simulink model "simulated_physical_reactor_v4_isolated"  (R2023a)
settings: Solver=FixedStepAuto  StartTime=0.0  StopTime=500  FixedStep=ts  RelTol=1e-3
values from neighbouring files (symbols this model uses):
  actionDelay = 10    [MainCode.m]
  buffer = 10    [MainCode.m]
  C0_attack_c = 0    [MainCode.m]
  C0_noise = 1    [MainCode.m]
  C0_post_attack = 0    [MainCode.m]
  C0_post_attack_val = -.25    (= -0.25)    [MainCode.m]
  Ccell0 = cell0 / v_cell    (= 15384.6153846)    [MainCode.m]
  CG0 = 185    [MainCode.m]
  CG_attack_c = 55    [MainCode.m]
  CG_attack_time = 175    [MainCode.m]
  CG_fake_failure = 0    [MainCode.m]
  CG_fake_failure_noise = 8    [MainCode.m]
  CG_increase_b = 0    [MainCode.m]
  CG_increase_rate = 2    [MainCode.m]
  cg_noGrowth = 10    [MainCode.m]
  CG_noise = 1    [MainCode.m]
  CG_post_attack = 1    [MainCode.m]
  CG_post_attack_val = .25    (= 0.25)    [MainCode.m]
  CG_ramp_attack = 1    [MainCode.m]
  CG_ramp_time = 125    [MainCode.m]
  CG_target = 50    [MainCode.m]
  CM = 4    [MainCode.m]
  CO0 = .245    (= 0.245)    [MainCode.m]
  CO_attack_time = 80    [MainCode.m]
  CO_fake_failure = 0    [MainCode.m]
  CO_fake_failure_mean = .08    (= 0.08)    [MainCode.m]
  CO_fake_failure_noise = .005    (= 0.005)    [MainCode.m]
  CO_ramp_attack = 0    [MainCode.m]
  CO_ramp_time = 100    [MainCode.m]
  count_thresh = 3    [MainCode.m]
  F_fresh_max = 25    [MainCode.m]
  F_net = F_fresh_start + F_recycle_start    (= 334.8)    [MainCode.m]
  flowrateNoiseActive = 0    [MainCode.m]
  flowrateNoiseVal = 0.5 / 100    (= 0.005)    [MainCode.m]
  fresh_attack = 0    [MainCode.m]
  fresh_attack_time = 70    [MainCode.m]
  fresh_attack_val = .1    (= 0.1)    [MainCode.m]
  freshPump_fail_time = 30    [MainCode.m]
  freshPump_failure = 0    [MainCode.m]
  freshPump_response_increases = 2    [MainCode.m]
  freshPump_response_window = 10    [MainCode.m]
  g_failure_start_t = 80    [MainCode.m]
  g_fault_wait_time = 10    [MainCode.m]
  g_flowrate_control_windowsize = 10    [MainCode.m]
  g_lownoise_val = 1.25    [MainCode.m]
  g_numpoints_fail = g_standdev_window_size+1    (= 16)    [MainCode.m]
  g_numpoints_low = 4    [MainCode.m]
  g_prob_arraylen = 15    [MainCode.m]
  g_prob_count = 6    [MainCode.m]
  g_prob_thresh = .45    (= 0.45)    [MainCode.m]
  g_standdev_window_size = 15    [MainCode.m]
  g_standev_tol = 7    [MainCode.m]
  glucose_fail_noise = 10    [MainCode.m]
  glucosesensor_failure = 0    [MainCode.m]
  lowConc_controller_onState = 1    [MainCode.m]
  mean_noise_C0 = 0    [MainCode.m]
  mean_noise_CG = 0    [MainCode.m]
  mu_max = 0.0251    [MainCode.m]
  n_size = t_window/ts    (= 2.5)    [MainCode.m]
  n_size_CG = n_size    (= 2.5)    [MainCode.m]
  o2_alpha = .20    (= 0.2)    [MainCode.m]
  o2_fail_mean = .008    (= 0.008)    [MainCode.m]
  o2_fail_noise = .005    (= 0.005)    [MainCode.m]
  o2_fail_time = 50    [MainCode.m]
  o2_fault_halfrange = .01    (= 0.01)    [MainCode.m]
  o2_fault_numpoints = 5    [MainCode.m]
  o2_lownoise_val = .0008    (= 0.0008)    [MainCode.m]
  o2_movingaverage_window = 10    [MainCode.m]
  o2_numpoints_low = 6    [MainCode.m]
  o2_prob_arraylen = 10    [MainCode.m]
  o2_prob_count = 6    [MainCode.m]
  o2_prob_thresh = .45    (= 0.45)    [MainCode.m]
  o2sensor_failure = 0    [MainCode.m]
  OCR = 2.8e-11    [MainCode.m]
  p_thresh = .4    (= 0.4)    [MainCode.m]
  rec_attack = 0    [MainCode.m]
  rec_attack_time = 50    [MainCode.m]
  rec_attack_val = 120    [MainCode.m]
  recPump_drop_val = .02    (= 0.02)    [MainCode.m]
  recPump_fail_time = 30    [MainCode.m]
  recPump_failure = 0    [MainCode.m]
  recPump_rollingavg_samples_buildup = 10    [MainCode.m]
  recPump_smallDrop_size = 0.006    [MainCode.m]
  stdev_noise_C0 = .002    (= 0.002)    [MainCode.m]
  stdev_noise_CG = 3.5    [MainCode.m]
  t_crit_CG = .7    (= 0.7)    [MainCode.m]
  ts = 1    [MainCode.m]
  V = 65.0    (= 65)    [MainCode.m]
  v_cell = 65    [MainCode.m]
  YGC = 155 * 10^-6    (= 0.000155)    [MainCode.m]
undefined symbols (not defined in the file or in its folder): DiscIntNeverNeededParam, recPump_numDrops_waitTime, recPump_rollingavg_numDrops
libraries: simulink x16, sldrtlib x11, dspstat3 x8, aerolibanimutils x1
(part 2 of 3)

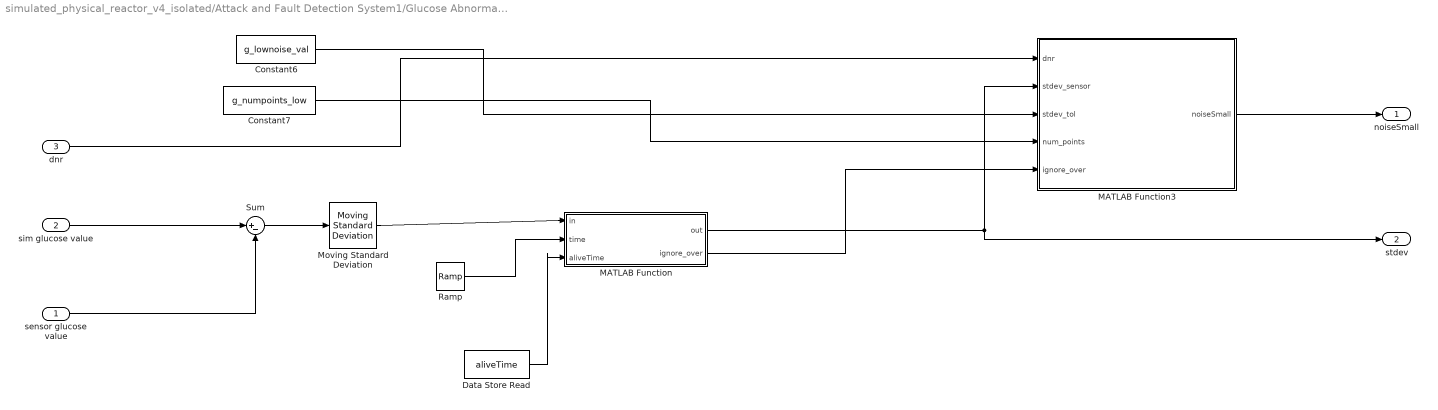
== system simulated_physical_reactor_v4_isolated/Attack and Fault Detection System1/Glucose Abnormally Low Noise Detection ==
  sensor glucose value : Inport
  sim glucose value : Inport  Port=2
  dnr : Inport  Port=3
  Constant6 : Constant  Value=g_lownoise_val
  Constant7 : Constant  Value=g_numpoints_low
  Data Store Read : DataStoreRead  DataStoreName=aliveTime  IndexOptions=Index vector (dialog)  Indices=1  OutputSizes=1
  MATLAB Function : MATLAB Function  TreatAsAtomicUnit=on
  MATLAB Function3 : MATLAB Function  TreatAsAtomicUnit=on
  Moving Standard Deviation : dspstat3/Moving Standard Deviation  Method=Sliding window  ForgettingFactorPort=off  SpecifyWindowLength=on  WindowLength=g_standdev_window_size  OverlapLength=g_standdev_window_size-1  AllowArbitraryInputLength=off  ForgettingFactor=0.9  SimulateUsing=Code generation
  Ramp : simulink/Sources/Ramp  slope=1  start=0  InitialOutput=0
  Sum : Sum  Inputs=|+-
  noiseSmall : Outport
  stdev : Outport  Port=2
  wires:
  MATLAB Function3/1(noiseSmall) -> noiseSmall/1
  Sum/1 -> Moving Standard Deviation/1
  Moving Standard Deviation/1 -> MATLAB Function/1(in)
  Ramp/1 -> MATLAB Function/2(time)
  sim glucose value/1 -> Sum/1
  MATLAB Function/1(out) -> MATLAB Function3/2(stdev_sensor), stdev/1
  sensor glucose value/1 -> Sum/2
  Constant6/1 -> MATLAB Function3/3(stdev_tol)
  Constant7/1 -> MATLAB Function3/4(num_points)
  MATLAB Function/2(ignore_over) -> MATLAB Function3/5(ignore_over)
  dnr/1 -> MATLAB Function3/1(dnr)
  Data Store Read/1 -> MATLAB Function/3(aliveTime)

== system simulated_physical_reactor_v4_isolated/Attack and Fault Detection System1/Glucose Deviation Detection ==
  Simulated g value : Inport
  Sensor g value : Inport  Port=2
  dnr : Inport  Port=3
  Constant : Constant  Value=g_prob_arraylen
  Constant1 : Constant  Value=g_prob_thresh
  Constant2 : Constant  Value=g_prob_count
  MATLAB Function : MATLAB Function  TreatAsAtomicUnit=on
  MATLAB Function1 : MATLAB Function  TreatAsAtomicUnit=on
  Moving Standard Deviation : dspstat3/Moving Standard Deviation  Method=Sliding window  ForgettingFactorPort=off  SpecifyWindowLength=on  WindowLength=g_standdev_window_size  OverlapLength=g_standdev_window_size-1  AllowArbitraryInputLength=off  ForgettingFactor=0.9  SimulateUsing=Code generation
  Sum : Sum  Inputs=|+-
  isDeviated : Outport
  likelihood : Outport  Port=2
  wires:
  Moving Standard Deviation/1 -> MATLAB Function/3(std_dev)
  MATLAB Function/1(likelihood) -> likelihood/1, MATLAB Function1/2(prob)
  Simulated g value/1 -> Sum/2
  Constant/1 -> MATLAB Function/4(g_prob_arraylen)
  Sensor g value/1 -> Moving Standard Deviation/1, Sum/1
  Sum/1 -> MATLAB Function/2(new_sens_value)
  MATLAB Function1/1(isDeviated) -> isDeviated/1
  Constant1/1 -> MATLAB Function1/3(thresh)
  Constant2/1 -> MATLAB Function1/4(thresh_count)
  dnr/1 -> MATLAB Function1/1(dnr), MATLAB Function/1(dnr)

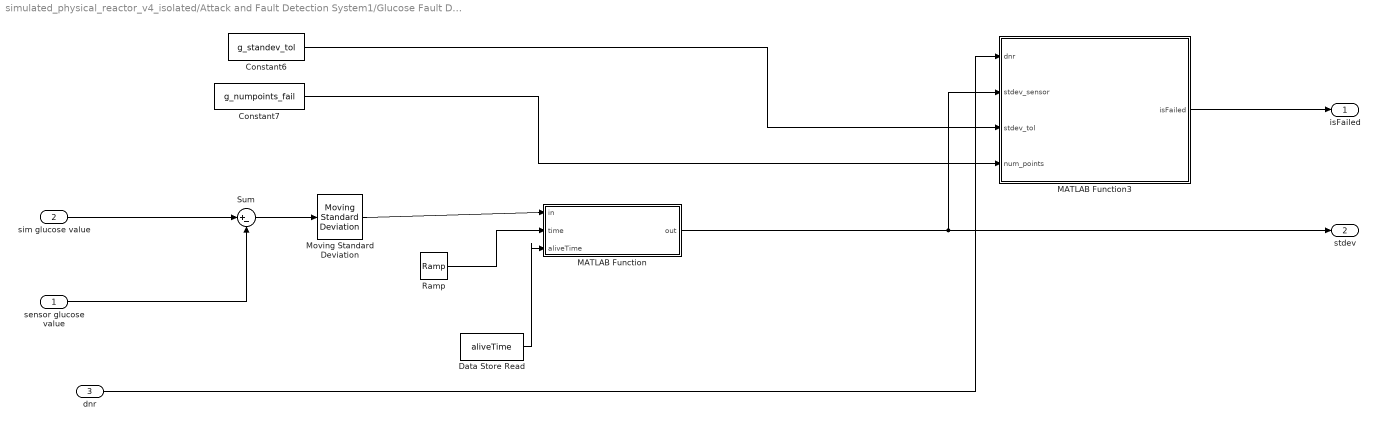
== system simulated_physical_reactor_v4_isolated/Attack and Fault Detection System1/Glucose Fault Detection ==
  sensor glucose value : Inport
  sim glucose value : Inport  Port=2
  dnr : Inport  Port=3
  Constant6 : Constant  Value=g_standev_tol
  Constant7 : Constant  Value=g_numpoints_fail
  Data Store Read : DataStoreRead  DataStoreName=aliveTime  IndexOptions=Index vector (dialog)  Indices=1  OutputSizes=1
  MATLAB Function : MATLAB Function  TreatAsAtomicUnit=on
  MATLAB Function3 : MATLAB Function  TreatAsAtomicUnit=on
  Moving Standard Deviation : dspstat3/Moving Standard Deviation  Method=Sliding window  ForgettingFactorPort=off  SpecifyWindowLength=on  WindowLength=g_standdev_window_size  OverlapLength=g_standdev_window_size-1  AllowArbitraryInputLength=off  ForgettingFactor=0.9  SimulateUsing=Code generation
  Ramp : simulink/Sources/Ramp  slope=1  start=0  InitialOutput=0
  Sum : Sum  Inputs=|+-
  isFailed : Outport
  stdev : Outport  Port=2
  wires:
  sim glucose value/1 -> Sum/1
  sensor glucose value/1 -> Sum/2
  MATLAB Function/1(out) -> stdev/1, MATLAB Function3/2(stdev_sensor)
  Sum/1 -> Moving Standard Deviation/1
  Moving Standard Deviation/1 -> MATLAB Function/1(in)
  Constant7/1 -> MATLAB Function3/4(num_points)
  Constant6/1 -> MATLAB Function3/3(stdev_tol)
  Ramp/1 -> MATLAB Function/2(time)
  MATLAB Function3/1(isFailed) -> isFailed/1
  dnr/1 -> MATLAB Function3/1(dnr)
  Data Store Read/1 -> MATLAB Function/3(aliveTime)

== system simulated_physical_reactor_v4_isolated/Attack and Fault Detection System1/Oxygen Abnormally Low Noise Detection1 ==
  sensor o2 value : Inport
  sim o2 value : Inport  Port=2
  dnr : Inport  Port=3
  Constant6 : Constant  Value=o2_lownoise_val
  Constant7 : Constant  Value=o2_numpoints_low
  Data Store Read : DataStoreRead  DataStoreName=aliveTime  IndexOptions=Index vector (dialog)  Indices=1  OutputSizes=1
  MATLAB Function : MATLAB Function  TreatAsAtomicUnit=on
  MATLAB Function3 : MATLAB Function  TreatAsAtomicUnit=on
  Moving Standard Deviation : dspstat3/Moving Standard Deviation  Method=Sliding window  ForgettingFactorPort=off  SpecifyWindowLength=on  WindowLength=g_standdev_window_size  OverlapLength=g_standdev_window_size-1  AllowArbitraryInputLength=off  ForgettingFactor=0.9  SimulateUsing=Code generation
  Ramp : simulink/Sources/Ramp  slope=1  start=0  InitialOutput=0
  Sum : Sum  Inputs=|+-
  noiseSmall : Outport
  stdev : Outport  Port=2
  wires:
  MATLAB Function3/1(noiseSmall) -> noiseSmall/1
  Sum/1 -> Moving Standard Deviation/1
  Moving Standard Deviation/1 -> MATLAB Function/1(in)
  Ramp/1 -> MATLAB Function/2(time)
  sim o2 value/1 -> Sum/1
  MATLAB Function/1(out) -> MATLAB Function3/2(stdev_sensor), stdev/1
  sensor o2 value/1 -> Sum/2
  Constant6/1 -> MATLAB Function3/3(stdev_tol)
  Constant7/1 -> MATLAB Function3/4(num_points)
  MATLAB Function/2(ignore_over) -> MATLAB Function3/5(ignore_over)
  dnr/1 -> MATLAB Function3/1(dnr)
  Data Store Read/1 -> MATLAB Function/3(aliveTime)

== system simulated_physical_reactor_v4_isolated/Attack and Fault Detection System1/Oxygen Deviation Detection1 ==
  Simulated o2 value : Inport
  Sensor o2 value : Inport  Port=2
  dnr : Inport  Port=3
  Constant : Constant  Value=o2_prob_arraylen
  Constant1 : Constant  Value=o2_prob_thresh
  Constant2 : Constant  Value=o2_prob_count
  MATLAB Function : MATLAB Function  TreatAsAtomicUnit=on
  MATLAB Function1 : MATLAB Function  TreatAsAtomicUnit=on
  Moving Standard Deviation : dspstat3/Moving Standard Deviation  Method=Sliding window  ForgettingFactorPort=off  SpecifyWindowLength=on  WindowLength=g_standdev_window_size  OverlapLength=g_standdev_window_size-1  AllowArbitraryInputLength=off  ForgettingFactor=0.9  SimulateUsing=Code generation
  Sum : Sum  Inputs=|+-
  isDeviated : Outport
  likelihood : Outport  Port=2
  wires:
  Moving Standard Deviation/1 -> MATLAB Function/3(std_dev)
  MATLAB Function/1(likelihood) -> likelihood/1, MATLAB Function1/2(prob)
  Simulated o2 value/1 -> Sum/2
  Constant/1 -> MATLAB Function/4(o2_prob_arraylen)
  Sensor o2 value/1 -> Moving Standard Deviation/1, Sum/1
  Sum/1 -> MATLAB Function/2(new_sens_value)
  MATLAB Function1/1(isDeviated) -> isDeviated/1
  Constant1/1 -> MATLAB Function1/3(thresh)
  Constant2/1 -> MATLAB Function1/4(thresh_count)
  dnr/1 -> MATLAB Function1/1(dnr), MATLAB Function/1(dnr)

== system simulated_physical_reactor_v4_isolated/Attack and Fault Detection System1/Oxygen Sensor Failure Detection ==
  o2_sensor : Inport
  dnr : Inport  Port=2
  Constant : Constant  Value=o2_fail_mean
  Constant2 : Constant  Value=o2_fault_halfrange
  Constant3 : Constant  Value=o2_fault_numpoints
  MATLAB Function : MATLAB Function  TreatAsAtomicUnit=on
  MATLAB Function1 : MATLAB Function  TreatAsAtomicUnit=on
  MATLAB Function2 : MATLAB Function  TreatAsAtomicUnit=on
  isFailed : Outport
  o2Distrubed : Outport  Port=2
  wires:
  Constant2/1 -> MATLAB Function2/4(half_range)
  Constant3/1 -> MATLAB Function2/5(num_points)
  Constant/1 -> MATLAB Function2/3(fail_val)
  o2_sensor/1 -> MATLAB Function2/2(o2_sensor)
  MATLAB Function2/1(isFailed) -> MATLAB Function/5(isFailed_begin), MATLAB Function1/1(isFailed)
  MATLAB Function1/1(o2_fault) -> isFailed/1
  MATLAB Function1/2(o2_disturb) -> o2Distrubed/1
  MATLAB Function/1(isFlat) -> MATLAB Function1/2(isFlat)
  dnr/1 -> MATLAB Function2/1(dnr)

== system simulated_physical_reactor_v4_isolated/Attack and Fault Detection System1/Recycle Pump Fault Detection ==
  oxygen sensor : Inport
  dnr : Inport  Port=2
  net flowrate commanded : Inport  Port=3
  Constant : Constant  Value=recPump_drop_val
  Constant1 : Constant  Value=recPump_numDrops_waitTime
  Constant2 : Constant  Value=recPump_rollingavg_numDrops
  Constant3 : Constant  Value=recPump_rollingavg_samples_buildup
  Constant4 : Constant  Value=recPump_smallDrop_size
  MATLAB Function : MATLAB Function  TreatAsAtomicUnit=on
  noRecycleResponse : Outport
  delta_o2 : Outport  Port=2
  rolling_avg_o2 : Outport  Port=3
  wires:
  net flowrate commanded/1 -> MATLAB Function/2(new_flowrate_commanded)
  MATLAB Function/1(RecyclePumpFail) -> noRecycleResponse/1
  oxygen sensor/1 -> MATLAB Function/3(oxygen_sensor)
  Constant/1 -> MATLAB Function/8(large_drop_val)
  Constant1/1 -> MATLAB Function/6(rolling_avg_samples_wait)
  Constant4/1 -> MATLAB Function/7(o2_rollavg_drop_spec)
  Constant2/1 -> MATLAB Function/5(numDrops)
  Constant3/1 -> MATLAB Function/4(samples_to_wait)
  MATLAB Function/2(delta_o2_out) -> delta_o2/1
  MATLAB Function/3(rolling_avg_out) -> rolling_avg_o2/1
  dnr/1 -> MATLAB Function/1(dnr)

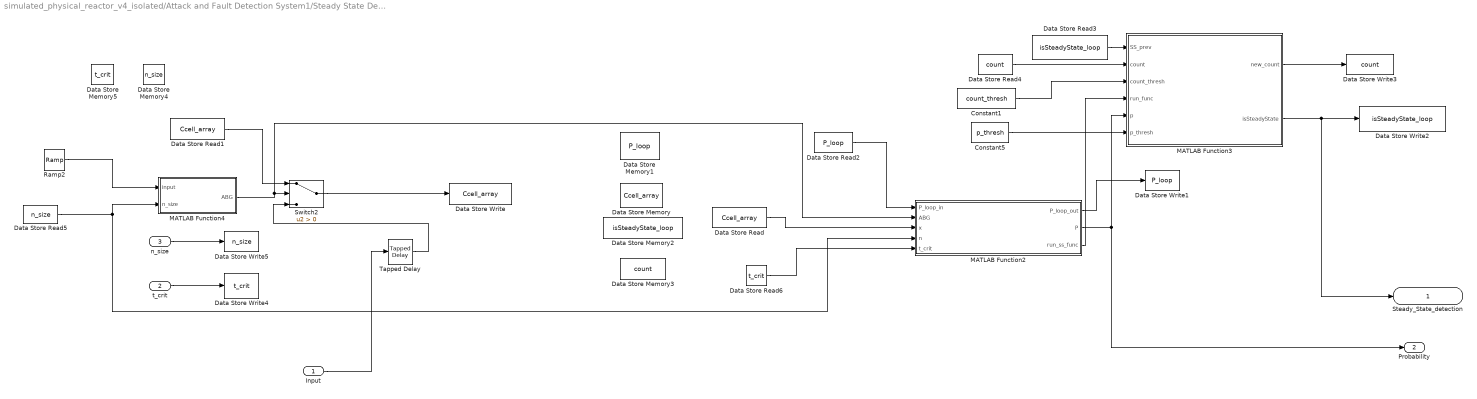
== system simulated_physical_reactor_v4_isolated/Attack and Fault Detection System1/Steady State Detection System1 ==
  Input : Inport
  t_crit : Inport  Port=2
  n_size : Inport  Port=3
  Constant1 : Constant  Value=count_thresh
  Constant5 : Constant  Value=p_thresh
  Data Store Memory : DataStoreMemory  DataStoreName=Ccell_array  ReadBeforeWriteMsg=warning  WriteAfterWriteMsg=warning  WriteAfterReadMsg=warning  InitialValue=zeros(1,n_size)  ShowAdditionalParam=off  OutDataTypeStr=double
  Data Store Memory1 : DataStoreMemory  DataStoreName=P_loop  ReadBeforeWriteMsg=warning  WriteAfterWriteMsg=warning  WriteAfterReadMsg=warning  ShowAdditionalParam=off
  Data Store Memory2 : DataStoreMemory  DataStoreName=isSteadyState_loop  ReadBeforeWriteMsg=warning  WriteAfterWriteMsg=warning  WriteAfterReadMsg=warning  ShowAdditionalParam=off
  Data Store Memory3 : DataStoreMemory  DataStoreName=count  ReadBeforeWriteMsg=warning  WriteAfterWriteMsg=warning  WriteAfterReadMsg=warning  ShowAdditionalParam=off
  Data Store Memory4 : DataStoreMemory  DataStoreName=n_size  ReadBeforeWriteMsg=warning  WriteAfterWriteMsg=warning  WriteAfterReadMsg=warning  ShowAdditionalParam=off
  Data Store Memory5 : DataStoreMemory  DataStoreName=t_crit  ReadBeforeWriteMsg=warning  WriteAfterWriteMsg=warning  WriteAfterReadMsg=warning  ShowAdditionalParam=off
  Data Store Read : DataStoreRead  DataStoreName=Ccell_array  IndexOptions=Index vector (dialog)  Indices=1  OutputSizes=1
  Data Store Read1 : DataStoreRead  DataStoreName=Ccell_array  IndexOptions=Index vector (dialog)  Indices=1  OutputSizes=1
  Data Store Read2 : DataStoreRead  DataStoreName=P_loop  IndexOptions=Index vector (dialog)  Indices=1  OutputSizes=1
  Data Store Read3 : DataStoreRead  DataStoreName=isSteadyState_loop  IndexOptions=Index vector (dialog)  Indices=1  OutputSizes=1
  Data Store Read4 : DataStoreRead  DataStoreName=count  IndexOptions=Index vector (dialog)  Indices=1  OutputSizes=1
  Data Store Read5 : DataStoreRead  DataStoreName=n_size  IndexOptions=Index vector (dialog)  Indices=1  OutputSizes=1
  Data Store Read6 : DataStoreRead  DataStoreName=t_crit  IndexOptions=Index vector (dialog)  Indices=1  OutputSizes=1
  Data Store Write : DataStoreWrite  DataStoreName=Ccell_array  IndexOptions=Index vector (dialog)  Indices=1  OutputSizes=1
  Data Store Write1 : DataStoreWrite  DataStoreName=P_loop  IndexOptions=Index vector (dialog)  Indices=1  OutputSizes=1
  Data Store Write2 : DataStoreWrite  DataStoreName=isSteadyState_loop  IndexOptions=Index vector (dialog)  Indices=1  OutputSizes=1
  Data Store Write3 : DataStoreWrite  DataStoreName=count  IndexOptions=Index vector (dialog)  Indices=1  OutputSizes=1
  Data Store Write4 : DataStoreWrite  DataStoreName=t_crit  IndexOptions=Index vector (dialog)  Indices=1  OutputSizes=1
  Data Store Write5 : DataStoreWrite  DataStoreName=n_size  IndexOptions=Index vector (dialog)  Indices=1  OutputSizes=1
  MATLAB Function2 : MATLAB Function  TreatAsAtomicUnit=on
  MATLAB Function3 : MATLAB Function  TreatAsAtomicUnit=on
  MATLAB Function4 : MATLAB Function  TreatAsAtomicUnit=on
  Ramp2 : simulink/Sources/Ramp  slope=1/ts  start=0  InitialOutput=0
  Switch2 : Switch  Criteria=u2 > Threshold  SaturateOnIntegerOverflow=off  InputSameDT=off
  Tapped Delay : simulink/Discrete/Tapped Delay  vinit=0.0  samptime=-1  NumDelays=n_size  DelayOrder=Oldest  includeCurrent=off
  Steady_State_detection : Outport
  Probability : Outport  Port=2
  wires:
  MATLAB Function3/2(isSteadyState) -> Steady_State_detection/1, Data Store Write2/1
  MATLAB Function2/1(P_loop_out) -> Data Store Write1/1
  Data Store Read2/1 -> MATLAB Function2/1(P_loop_in)
  Input/1 -> Tapped Delay/1
  Data Store Read4/1 -> MATLAB Function3/2(count)
  Data Store Read1/1 -> Switch2/1
  MATLAB Function2/2(P) -> Probability/1, MATLAB Function3/5(p)
  Constant5/1 -> MATLAB Function3/6(p_thresh)
  Data Store Read5/1 -> MATLAB Function4/2(n_size), MATLAB Function2/4(n)
  MATLAB Function3/1(new_count) -> Data Store Write3/1
  Ramp2/1 -> MATLAB Function4/1(input)
  MATLAB Function4/1(ABG) -> MATLAB Function2/2(ABG), Switch2/2
  Tapped Delay/1 -> Switch2/3
  Data Store Read6/1 -> MATLAB Function2/5(t_crit)
  t_crit/1 -> Data Store Write4/1
  n_size/1 -> Data Store Write5/1
  Data Store Read/1 -> MATLAB Function2/3(x)
  Switch2/1 -> Data Store Write/1
  MATLAB Function2/3(run_ss_func) -> MATLAB Function3/4(run_func)
  Data Store Read3/1 -> MATLAB Function3/1(SS_prev)
  Constant1/1 -> MATLAB Function3/3(count_thresh)

== matlab function simulated_physical_reactor_v4_isolated/Oxygen sensor failure/MATLAB Function ==
  data: o2_in input; o2_out output; o2_noise input; o2_const input; isFailed input; o2_fail_time input; time input
function o2_out = o2_failure(o2_in, o2_noise, o2_const, isFailed, o2_fail_time,time)

if (isFailed == 1 && time>o2_fail_time)
    o2_out = normrnd(o2_const,o2_noise);
else
    o2_out = o2_in;
end

== matlab function simulated_physical_reactor_v4_isolated/Attack Response System/Prevents net flowrate from decreasing ==
  data: F_re_in input; F_fr_in input; F_re_out output; Fnet input; F_fr_out output; controllerAction input
function [F_re_out, F_fr_out] = minRate(F_re_in, F_fr_in, Fnet, controllerAction)

%total flowrate
Fin_total = F_re_in + F_fr_in;

%compute flowrate ratio (as recycle percentage of total flowrate)
recycle_percentage = F_re_in / Fin_total; 

%if controller is on and Fnet is exceeded, allow control actions but
%preserve ratio
if (Fin_total<Fnet && controllerAction==1)
    F_re_out = recycle_percentage * Fnet;
    F_fr_out = Fnet - F_re_out;
else
    F_re_out = F_re_in;
    F_fr_out = F_fr_in;
end

== matlab function simulated_physical_reactor_v4_isolated/Flowrate Inconsistency System/MATLAB Function ==
  data: input_flowrate input; output_flowrate output; noise_percentage input; isActive input
function output_flowrate = flowrateNoise(input_flowrate, noise_percentage, isActive)

if isActive==false
    noise = 0;
else %isActive is true
    noise = normrnd(0, input_flowrate) * noise_percentage;
end

output_flowrate = input_flowrate + noise;

== matlab function simulated_physical_reactor_v4_isolated/Simulation Failsafe Process Control Adjustment1/Glucose flow increaser1 ==
  data: C_target input; F_fresh_new output; C_actual input; F_fresh_max input; f_fresh_in input; f_recycle_in input; F_net input; F_recycle_new output; time input; CG_increase_rate input; CG_increase_b input; time_mem_in input; time_mem_out output; controllerOnstate input; buffer input
function [F_fresh_new, F_recycle_new, time_mem_out]  = FlowIncrease(C_target, C_actual,F_fresh_max, f_fresh_in, f_recycle_in, F_net, time,CG_increase_rate,CG_increase_b, time_mem_in, controllerOnstate, buffer)

total_flowin = f_recycle_in+f_fresh_in;

%only run if sensor should be considered and target is low
if ((C_actual < C_target) && controllerOnstate==1 && ((time+5)>time_mem_in) && (time>buffer))
    F_fresh_new = CG_increase_rate*f_fresh_in + CG_increase_b;
    F_recycle_new = total_flowin - F_fresh_new;
    time_mem_out = time;
else
    F_fresh_new = f_fresh_in;
    F_recycle_new = f_recycle_in;
    time_mem_out = time_mem_in;
end

if (F_fresh_new>=F_fresh_max)
    F_fresh_new = F_fresh_max;
    F_recycle_new = (F_net - F_fresh_max);
end

== matlab function simulated_physical_reactor_v4_isolated/Attack Response System/Prevents flowrate ratio from decreasing ==
  data: F_re_in input; F_fr_in input; recycle_percent_mem_in input; controllerAction input; F_re_out output; F_fr_out output; recycle_percent_mem_out output
function [F_re_out, F_fr_out, recycle_percent_mem_out] = ratioIncreaser(F_re_in, F_fr_in, recycle_percent_mem_in, controllerAction)


%total flowrate
Fin_total = F_re_in + F_fr_in;

%compute flowrate ratio (as recycle percentage of total flowrate)
in_recycle_percentage = F_re_in / Fin_total; 

lower_perc = min(in_recycle_percentage, recycle_percent_mem_in);

%if controller is on, prevent percentage from increasing
if (controllerAction==1)
    recycle_percent_mem_out = lower_perc;
    F_re_out = recycle_percent_mem_out * F_re_in;
    F_fr_out = Fin_total - F_re_out;
else
    recycle_percent_mem_out =  recycle_percent_mem_in;
    F_re_out = F_re_in;
    F_fr_out = F_fr_in;
end

== matlab function simulated_physical_reactor_v4_isolated/Compromised Sensor Action System/MATLAB Function1 ==
  data: number input; ignoreSensor output
function ignoreSensor = containsTwoOrSix(number)

% Convert number to string for easier manipulation
num_str = sprintf('%d', int64(number));

% Check if real glucose sensor should be ignored
if contains(num_str, '2') || contains(num_str, '6')
    ignoreSensor = 1;
else
    ignoreSensor = 0;
end

== matlab function simulated_physical_reactor_v4_isolated/Regular Process Control Adjustment/Glucose flow increaser1 ==
  data: C_target input; F_fresh_new output; C_actual input; F_fresh_max input; f_fresh_in input; f_recycle_in input; F_net input; F_recycle_new output; time input; CG_increase_rate input; CG_increase_b input; time_mem_in input; time_mem_out output; controllerOnstate input; buffer input; actionDelay input
function [F_fresh_new, F_recycle_new, time_mem_out]  = FlowIncrease(C_target, C_actual,F_fresh_max, f_fresh_in, f_recycle_in, F_net, time,CG_increase_rate,CG_increase_b, time_mem_in, controllerOnstate, buffer, actionDelay)

total_flowin = f_recycle_in+f_fresh_in;

%only run if sensor should be considered and target is low
if ((C_actual < C_target) && controllerOnstate==1 && ((time-actionDelay)>time_mem_in) && (time>buffer))
    F_fresh_new = CG_increase_rate*f_fresh_in + CG_increase_b;
    F_recycle_new = total_flowin - F_fresh_new;
    time_mem_out = time;
else
    F_fresh_new = f_fresh_in;
    F_recycle_new = f_recycle_in;
    time_mem_out = time_mem_in;
end

if (F_fresh_new>=F_fresh_max)
    F_fresh_new = F_fresh_max;
    F_recycle_new = (F_net - F_fresh_max);
end

== matlab function simulated_physical_reactor_v4_isolated/Subsystem2/MATLAB Function1 ==
  data: u input; y output; alpha input
function y = ewma(u, alpha)
    persistent prev_ewma;
    if isempty(prev_ewma)
        prev_ewma = u;
    end
    
    % Calculate exponentially weighted moving average
    ewma = alpha * u + (1 - alpha) * prev_ewma;
    
    % Update the previous EWMA for the next iteration
    prev_ewma = ewma;
    
    y = ewma;
end

== matlab function simulated_physical_reactor_v4_isolated/CG Sensor Noise System/MATLAB Function6 ==
  data: mean input; std input; C input; C_noisy output
function C_noisy = fcn(mean, std, C)

r = normrnd(mean,std);

C_noisy = C + r;

== matlab function simulated_physical_reactor_v4_isolated/CG Attack System/MATLAB Function7 ==
  data: time input; in input; out output; attackval input; attackC input; attackTime input
function out = addAttack(time, in,attackval, attackC, attackTime)

if time > attackTime
    out = attackval*in + attackC + in;
else
    out = in;
end

== matlab function simulated_physical_reactor_v4_isolated/Simulated Reactor/MATLAB Function1 ==
  data: in input; out output
function out = notZero(in)

if in>0
    out=in;
else % in<0
    out = 0;
end

== matlab function simulated_physical_reactor_v4_isolated/Compromised Sensor Action System/MATLAB Function ==
  data: sim_fresh input; rec_out output; actual_fresh input; sim_rec input; actual_rec input; fresh_out output; ignoreSensor input
function [rec_out, fresh_out] = chooseGreater(sim_fresh, actual_fresh, sim_rec, actual_rec, ignoreSensor)


if ignoreSensor==1
    fresh_out = sim_fresh;
    rec_out = sim_rec;
else %sim_fresh<=actual_fresh
    fresh_out = actual_fresh;
    rec_out = actual_rec;
end

== matlab function simulated_physical_reactor_v4_isolated/Simulated Reactor/MATLAB Function2 ==
  data: statement input; num output
function num = tf_num(statement)

if statement==true
    num = 1;
else
    num = 0;
end

== matlab function simulated_physical_reactor_v4_isolated/Subsystem2/MATLAB Function ==
  data: inlet_o2_conc input; cell_count output; exit_o2_actual_conc input; exit_o2_sim_conc input; faultCode input; dt input; OCR input; flowrate input; window_wait input; time input
function cell_count = fcn(inlet_o2_conc, exit_o2_actual_conc, exit_o2_sim_conc, faultCode, dt, OCR, flowrate, window_wait, time)

% Convert number to string for easier manipulation
num_str = sprintf('%d', int64(faultCode));

% Check if '1' or '5' is present in the number
if contains(num_str, '1') || contains(num_str, '5')
    sensorFault = 1;
else
    sensorFault = 0;
end


if sensorFault==0
    exit_o2_conc = exit_o2_actual_conc;
else %sensor fault/compromised
    exit_o2_conc = exit_o2_sim_conc;
end


dCO = inlet_o2_conc - exit_o2_conc;
delta_o2_amount = dCO * flowrate * dt / 1000;


%o2_enter_amount = inlet_o2_conc * flowrate  * dt / 1000; %mmol during dt
%o2_exit_amount = exit_o2_conc * flowrate * dt / 1000;

%amount of o2 consumed in reactor 
%delta_o2_amount = o2_enter_amount - o2_exit_amount; %mmol during dt

%OCR: mmol o2 / (cell * hour)
cell_count = delta_o2_amount / (OCR * dt);

%generate no prediction while the moving average is working in
if time<window_wait || cell_count<0
    cell_count=0;
end

== matlab function simulated_physical_reactor_v4_isolated/CO Sensor Noise System/MATLAB Function14 ==
  data: mean input; std input; C input; C_noisy output
function C_noisy = fcn(mean, std, C)

r = normrnd(mean,std);

C_noisy = C + r;

== matlab function simulated_physical_reactor_v4_isolated/Attack Response System/Prevents net flowrate from increasing ==
  data: F_re_in input; F_fr_in input; F_re_out output; Fnet input; F_fr_out output; controllerAction input
function [F_re_out, F_fr_out] = maxRate(F_re_in, F_fr_in, Fnet, controllerAction)

%total flowrate
Fin_total = F_re_in + F_fr_in;

%compute flowrate ratio (as recycle percentage of total flowrate)
recycle_percentage = F_re_in / Fin_total; 

%if controller is on and Fnet is exceeded, allow control actions but
%preserve ratio
if (Fin_total>Fnet && controllerAction==1)
    F_re_out = recycle_percentage * Fnet;
    F_fr_out = Fnet - F_re_out;
else
    F_re_out = F_re_in;
    F_fr_out = F_fr_in;
end

== matlab function simulated_physical_reactor_v4_isolated/CG Attack System/MATLAB Function ==
  data: ramp_attack_trigger input; attack_val output; ramp_time input; time input; attack_time input; c_attack_val input; attack_const input; attack_c output
function [attack_val, attack_c] = fcn(ramp_attack_trigger, ramp_time, time, attack_time, c_attack_val, attack_const)

if (ramp_attack_trigger==0 || time<attack_time)
    attack_val = c_attack_val;
    attack_c = attack_const;
else %ramp attack is triggered AND time>attack_time
    attack_val = ((time-attack_time)/ramp_time) * c_attack_val;
    attack_c = ((time-attack_time)/ramp_time) * attack_const;
    if (time > (ramp_time + attack_time))
        attack_val = c_attack_val;
        attack_c = attack_const;
    end
end

== matlab function simulated_physical_reactor_v4_isolated/CG Attack System/MATLAB Function1 ==
  data: glucose_in input; glucoseOut output; glucose_noise input; isFailed input
function glucoseOut = glucose_failure(glucose_in, glucose_noise, isFailed)

if isFailed == 0
    glucoseOut = glucose_in;
else
    r = normrnd(0,glucose_noise);
    glucoseOut = glucose_in + r;
end

== matlab function simulated_physical_reactor_v4_isolated/CO Attack System/MATLAB Function ==
  data: ramp_attack_trigger input; attack_val output; ramp_time input; time input; attack_time input; c_attack_val input; attack_const input; attack_c output
function [attack_val, attack_c] = fcn(ramp_attack_trigger, ramp_time, time, attack_time, c_attack_val, attack_const)

if (ramp_attack_trigger==0 || time<attack_time)
    attack_val = c_attack_val;
    attack_c = attack_const;
else %ramp attack is triggered AND time>attack_time
    attack_val = ((time-attack_time)/ramp_time) * c_attack_val;
    attack_c = ((time-attack_time)/ramp_time) * attack_const;
    if (time > (ramp_time + attack_time))
        attack_val = c_attack_val;
        attack_c = attack_const;
    end
end

== matlab function simulated_physical_reactor_v4_isolated/CO Attack System/MATLAB Function7 ==
  data: time input; in input; out output; attackval input; attackC input; attackTime input
function out = addAttack(time, in,attackval, attackC, attackTime)

if time > attackTime
    out = attackval*in + attackC + in;
else
    out = in;
end

== matlab function simulated_physical_reactor_v4_isolated/Simulated Reactor/MATLAB Function3 ==
  data: divide input; out output; mult input
function out = divideNotZero(divide, mult)

if divide==0
    out = 0;
else
    out = mult/divide;
end

== matlab function simulated_physical_reactor_v4_isolated/Fresh Flowrate Attack System/MATLAB Function ==
  data: flow_in input; flow_out output; attack_on input; attack_val input; attack_time input; time input
function flow_out = pumpAttack(flow_in, attack_on, attack_val, attack_time, time)

if (attack_on==1 && time>=attack_time)
    flow_out = attack_val;
else
    flow_out = flow_in;
end

== matlab function simulated_physical_reactor_v4_isolated/Attack Response System/MATLAB Function ==
  data: number input; controllerAction output
function controllerAction = containsSeven(number)
    % Convert number to string for easier manipulation
    num_str = sprintf('%d', int64(number));
    
    % Check if '7' is present in the number
    if contains(num_str, '7')
        controllerAction = 1;
    else
        controllerAction = 0;
    end
end

== matlab function simulated_physical_reactor_v4_isolated/Recycle Flowrate Attack System/MATLAB Function ==
  data: flow_in input; flow_out output; attack_on input; attack_val input; attack_time input; time input
function flow_out = pumpAttack(flow_in, attack_on, attack_val, attack_time, time)

if (attack_on==1 && time>=attack_time)
    flow_out = attack_val;
else
    flow_out = flow_in;
end

== matlab function simulated_physical_reactor_v4_isolated/Attack and Fault Detection System1/Fresh Pump Fault Detection/MATLAB Function ==
  data: dnr input; flowrate_commanded input; freshPumpFail output; glucose_sensor input; samples_to_wait input; samples_increase_in_window input
function freshPumpFail  = noFreshResponse(dnr, flowrate_commanded, glucose_sensor, samples_to_wait, samples_increase_in_window)

%%%%%%% initilizing memory variables
persistent prevFlowrate;
persistent wait_count;
persistent glucoseIncreasesCount;
persistent prevGlucose;
persistent isFailed;

if isempty(prevFlowrate)
    prevFlowrate = flowrate_commanded;
end

if isempty(glucoseIncreasesCount)
    glucoseIncreasesCount = 0;
end

if isempty(prevGlucose)
    prevGlucose = glucose_sensor;
end

if isempty(wait_count)
    wait_count = 0;
end

if isempty(isFailed)
    isFailed = 0;
end

%initialize prevFlowrate
%if prevFlowrate==0
%    prevFlowrate = flowrate_commanded;
%end
%%%%%% end initialization

if(dnr==0)

    if flowrate_commanded>prevFlowrate
        %start the counter
        wait_count = wait_count + 1;
    else
        %if the count hasn't started, and flowrate hasnt increased, keep all 0
        if wait_count==0
            wait_count = 0;
            glucoseIncreasesCount = 0;
            %if the count has started, check for glucose increase
        else
            %increase glucose check counts if it has increased
            if glucose_sensor>prevGlucose
                glucoseIncreasesCount = glucoseIncreasesCount + 1;
            end
            %increase wait counter
            wait_count = wait_count+1;
        end
    end

    %change flowrate increase
    prevFlowrate = flowrate_commanded;
    prevGlucose = glucose_sensor;

    %if we waited all samples and saw enough increases, all good, reset
    if (wait_count>=(samples_to_wait+1) || glucoseIncreasesCount>=samples_increase_in_window)
        %reset all counts
        wait_count = 0;
        glucoseIncreasesCount = 0;
        %if we waited all samples and did not see increases, throw fail flag
    elseif ((wait_count>=samples_to_wait) && (glucoseIncreasesCount<=samples_increase_in_window))
        isFailed = 1;
        glucoseIncreasesCount = samples_increase_in_window + 1;
        wait_count = samples_to_wait + 1;
    end

    if isFailed==1
        wait_count = samples_to_wait + 1;
        glucoseIncreasesCount = samples_increase_in_window + 1;
    end

    freshPumpFail = isFailed;

else
    freshPumpFail=0;
end

%debugging variables

== matlab function simulated_physical_reactor_v4_isolated/Attack and Fault Detection System1/Glucose Abnormally Low Noise Detection/MATLAB Function ==
  data: in input; out output; time input; ignore_over output; aliveTime input
function [out, ignore_over] = ignore15(in, time, aliveTime)

if time>(15+aliveTime)
    out = in;
    ignore_over = 1;
else
    out = 0;
    ignore_over = 0;
end

== matlab function simulated_physical_reactor_v4_isolated/Attack and Fault Detection System1/Glucose Abnormally Low Noise Detection/MATLAB Function3 ==
  data: dnr input; noiseSmall output; stdev_sensor input; stdev_tol input; num_points input; ignore_over input
function noiseSmall = detectGFailure(dnr, stdev_sensor, stdev_tol, num_points, ignore_over)

%create fail count variable
persistent count_g_low;
%fill it if full
if isempty(count_g_low)
    count_g_low = 0;
end

if (dnr==0)
    if count_g_low==num_points
        noiseSmall = 1;
    else
        if (stdev_sensor<=stdev_tol && ignore_over == 1)
            count_g_low = count_g_low + 1;
        else
            count_g_low = 0;
        end
        noiseSmall = 0;
    end
else
    noiseSmall=0;
end

== matlab function simulated_physical_reactor_v4_isolated/Attack and Fault Detection System1/Glucose Deviation Detection/MATLAB Function ==
  data: dnr input; new_sens_value input; likelihood output; std_dev input; g_prob_arraylen input
function likelihood  = compute_likelihood_rolling(dnr, new_sens_value, std_dev, g_prob_arraylen)

persistent sens_arr;
%fill it if full
if isempty(sens_arr)
    sens_arr = zeros(1, g_prob_arraylen);
end

if (dnr==0)
    %shift array one left and add new element
    shifted_arr = [sens_arr(2:end)];
    sens_arr = [shifted_arr, new_sens_value];

    %compute probability array using values, mean (true value), and stdev
    %.500 is 100%, 0 and 1 are 0%
    p = normcdf(sens_arr, 0, std_dev);
    %shift down to be around 0
    p = p-.5;
    %get net distance away from mean
    p = abs(p);

    %net likelihood is average of array
    likelihood = mean(p);

else
    likelihood=0;

end
end

== matlab function simulated_physical_reactor_v4_isolated/Attack and Fault Detection System1/Glucose Deviation Detection/MATLAB Function1 ==
  data: dnr input; prob input; isDeviated output; thresh input; thresh_count input
function isDeviated  = fcn(dnr, prob, thresh, thresh_count)

persistent g_count;

if isempty(g_count)
    g_count = 0;
end

if (dnr==0)
    if g_count>=thresh_count
        isDeviated = true;
    else
        isDeviated = false;
        if prob <= thresh
            g_count = 0;
        else %prob > thresh
            g_count = g_count+1;
        end
    end
else
    isDeviated=false;
end

== matlab function simulated_physical_reactor_v4_isolated/Attack and Fault Detection System1/Glucose Fault Detection/MATLAB Function ==
  data: in input; out output; time input; aliveTime input
function out = ignore15(in, time, aliveTime)

if time>(15 + aliveTime)
    out = in;
else
    out = 0;
end

== matlab function simulated_physical_reactor_v4_isolated/Simulated Reactor/MATLAB Function ==
  data: mu_max input; CM input; CG input; Ccell input; cgNoGrowth input; dCcell_dt output; ts input; CO input
function dCcell_dt  = monodEq(mu_max, CM,CG,Ccell, cgNoGrowth, ts, CO) %,volume, cgNo)


dCcell_dt = (mu_max * Ccell * CG) / (CG + CM) * ts;

if (dCcell_dt < 0 || CG<=cgNoGrowth || CO<=.01)
    dCcell_dt = 0;
end

%val = (CG * volume / 100) / Ccell;

%if (val < cgNo)
%    dCcell_dt = 0;
%end

== matlab function simulated_physical_reactor_v4_isolated/Attack and Fault Detection System1/Glucose Fault Detection/MATLAB Function3 ==
  data: dnr input; isFailed output; stdev_sensor input; stdev_tol input; num_points input
function isFailed = detectGFailure(dnr, stdev_sensor, stdev_tol, num_points)

%create fail count variable
persistent count_g_fail;
%fill it if full
if isempty(count_g_fail)
    count_g_fail = 0;
end

if (dnr==0)
    if count_g_fail==num_points
        isFailed = 1;
    else
        if (stdev_sensor>=stdev_tol)
            count_g_fail = count_g_fail + 1;
        else
            count_g_fail = 0;
        end
        isFailed = 0;
    end
else
    isFailed=0;
end

== matlab function simulated_physical_reactor_v4_isolated/Attack and Fault Detection System1/MATLAB Function2 ==
  data: isFailed input; glucoseFault output; noise_small input; isDeviated input; waitAfterFirst input; glucoseAttacked output; potentialFault output
function [glucoseFault, glucoseAttacked, potentialFault] = glucoseSensorDetection(isFailed, noise_small, isDeviated, waitAfterFirst)

persistent g_fault_wait;

if isempty(g_fault_wait)
    g_fault_wait = 0;
end

if (isFailed==0 && noise_small==0 && isDeviated==0)
    glucoseFault = 0;
    glucoseAttacked = 0;
    potentialFault = 0;
else %any are triggered
    g_fault_wait = g_fault_wait + 1;
    glucoseFault = 0;
    glucoseAttacked = 0;
    potentialFault = 1;
end

if (g_fault_wait>=waitAfterFirst)
    potentialFault = 1;
    %first, pure fault detection
    if (isFailed==1 && noise_small==0 && isDeviated==0)
        glucoseFault = 1;
        glucoseAttacked = 0;
    else %(isFailed==0 && (noise_small==1 || isDeviated==1))
        glucoseFault = 0;
        glucoseAttacked = 1;
    end
end

== matlab function simulated_physical_reactor_v4_isolated/Attack and Fault Detection System1/MATLAB Function3 ==
  data: isFailed input; oxygenFault output; noise_small input; isDeviated input; waitAfterFirst input; oxygenAttacked output; potentialFault output
function [oxygenFault, oxygenAttacked, potentialFault] = oxygenSensorDetection(isFailed, noise_small, isDeviated, waitAfterFirst)

persistent o2_fault_wait;

if isempty(o2_fault_wait)
    o2_fault_wait = 0;
end

if (isFailed==0 && noise_small==0 && isDeviated==0)
    oxygenFault = 0;
    oxygenAttacked = 0;
    potentialFault = 0;
else %any are triggered
    o2_fault_wait = o2_fault_wait + 1;
    oxygenFault = 0;
    oxygenAttacked = 0;
    potentialFault = 1;
end

if (o2_fault_wait>=waitAfterFirst)
    potentialFault = 1;
    %first, pure fault detection
    if (isFailed==1 && noise_small==0 && isDeviated==0)
        oxygenFault = 1;
        oxygenAttacked = 0;
    else %(isFailed==0 && (noise_small==1 || isDeviated==1))
        oxygenFault = 0;
        oxygenAttacked = 1;
    end
end

== matlab function simulated_physical_reactor_v4_isolated/Attack and Fault Detection System1/Oxygen Abnormally Low Noise Detection1/MATLAB Function ==
  data: in input; out output; time input; ignore_over output; aliveTime input
function [out, ignore_over] = ignore15(in, time, aliveTime)

if time>(15+aliveTime)
    out = in;
    ignore_over = 1;
else
    out = 0;
    ignore_over = 0;
end

== matlab function simulated_physical_reactor_v4_isolated/Attack and Fault Detection System1/Oxygen Abnormally Low Noise Detection1/MATLAB Function3 ==
  data: dnr input; noiseSmall output; stdev_sensor input; stdev_tol input; num_points input; ignore_over input
function noiseSmall = detectO2Failure(dnr, stdev_sensor, stdev_tol, num_points, ignore_over)

%create fail count variable
persistent count_o2_low;
%fill it if full
if isempty(count_o2_low)
    count_o2_low = 0;
end

if (dnr==0)
    if count_o2_low==num_points
        noiseSmall = 1;
    else
        if (stdev_sensor<=stdev_tol && ignore_over == 1)
            count_o2_low = count_o2_low + 1;
        else
            count_o2_low = 0;
        end
        noiseSmall = 0;
    end
else
    noiseSmall=0;
end

== matlab function simulated_physical_reactor_v4_isolated/Attack and Fault Detection System1/Oxygen Deviation Detection1/MATLAB Function ==
  data: dnr input; new_sens_value input; likelihood output; std_dev input; o2_prob_arraylen input
function likelihood  = compute_likelihood_rolling(dnr, new_sens_value, std_dev, o2_prob_arraylen)

persistent sens_arr_o2;
%fill it if full
if isempty(sens_arr_o2)
    sens_arr_o2 = zeros(1, o2_prob_arraylen);
end

if (dnr==0)

    %shift array one left and add new element
    shifted_arr = [sens_arr_o2(2:end)];
    sens_arr_o2 = [shifted_arr, new_sens_value];

    %compute probability array using values, mean (true value), and stdev
    %.500 is 100%, 0 and 1 are 0%
    p = normcdf(sens_arr_o2, 0, std_dev);
    %shift down to be around 0
    p = p-.5;
    %get net distance away from mean
    p = abs(p);

    %net likelihood is average of array
    likelihood = mean(p);

else
    likelihood=0;
end
end

== matlab function simulated_physical_reactor_v4_isolated/Attack and Fault Detection System1/Oxygen Deviation Detection1/MATLAB Function1 ==
  data: dnr input; prob input; isDeviated output; thresh input; thresh_count input
function isDeviated  = fcn(dnr, prob, thresh, thresh_count)

persistent g_count;

if isempty(g_count)
    g_count = 0;
end

if(dnr==0)

    if g_count>=thresh_count
        isDeviated = true;
    else
        isDeviated = false;
        if prob <= thresh
            g_count = 0;
        else %prob > thresh
            g_count = g_count+1;
        end
    end
else
    isDeviated=false;
end

== matlab function simulated_physical_reactor_v4_isolated/Attack and Fault Detection System1/Oxygen Sensor Failure Detection/MATLAB Function ==
  data: glucose_sensor input; initial_window_size input; isFlat output; window_size input; deviation_accepted input; isFailed_begin input
function isFlat = glucoseFlatline(glucose_sensor, initial_window_size, window_size, deviation_accepted, isFailed_begin)

persistent glucose_avg;
persistent count1;
persistent isFlat_pers;
persistent glucose_avg_hold;
persistent did_deviate;

%initialize persistents

if isempty(glucose_avg)
    glucose_avg = 0;
end

if isempty(did_deviate)
    did_deviate = 1;
end

if isempty(glucose_avg_hold)
    glucose_avg_hold = 0;
end

if isempty(count1)
    count1 = 0;
end

if isempty(isFlat_pers)
    isFlat_pers = 0;
end

%end initialize



if isFailed_begin==0
    isFlat_pers = 0;
else %failed trigger
    if count1==0
        glucose_avg = glucose_sensor;
    end
    if (count1<initial_window_size)
        glucose_avg = (glucose_avg + glucose_sensor) / 2;
        glucose_avg_hold = glucose_avg;
    end
    if (count1<(initial_window_size + window_size) && count1>=initial_window_size)
        glucose_avg = (glucose_avg + glucose_sensor) / 2;
        if glucose_avg>glucose_avg_hold+deviation_accepted || glucose_avg<glucose_avg_hold-deviation_accepted
            isFlat_pers = 0;
        else
            did_deviate = 0;
        end
    end
    if (count1>=(initial_window_size + window_size) && did_deviate==1)
        isFlat_pers = 1;
        count1 = (initial_window_size + window_size);
    end
    count1=count1+1;
end

isFlat = isFlat_pers;

== matlab function simulated_physical_reactor_v4_isolated/Attack and Fault Detection System1/Oxygen Sensor Failure Detection/MATLAB Function1 ==
  data: isFailed input; o2_fault output; isFlat input; wait_time input; o2_disturb output
function [o2_fault, o2_disturb] = fcn(isFailed, isFlat, wait_time)

persistent o2failed_wait;
persistent o2_fault_trigger;

if isempty(o2failed_wait)
    o2failed_wait = 0;
end

if isempty(o2_fault_trigger)
    o2_fault_trigger = 0;
end

%check for reported sensor failure
if isFailed==1
    %check to see if the window has passed
    if o2failed_wait>=wait_time
        %if glucose is still changing, throw fault code
        if isFlat==0
            o2_fault_trigger = 1;
        end
    end
    %increase wait counter
    o2failed_wait = o2failed_wait+1;
    %throw disturbance code
    o2_disturb = 1;
else %sensor not failed
    o2_fault_trigger=0;
    o2_disturb=0;
    %reset counter
    o2failed_wait=0;
end

o2_fault = o2_fault_trigger;

== matlab function simulated_physical_reactor_v4_isolated/Attack and Fault Detection System1/Oxygen Sensor Failure Detection/MATLAB Function2 ==
  data: dnr input; o2_sensor input; isFailed output; fail_val input; half_range input; num_points input
function isFailed = detectO2Failure(dnr, o2_sensor, fail_val, half_range, num_points)

persistent count_o2_fail;
if isempty(count_o2_fail)
    count_o2_fail = 0;
end

if (dnr==0)
    if count_o2_fail==num_points
        isFailed = 1;
    else
        if (o2_sensor < (fail_val + half_range) && o2_sensor > (fail_val + half_range))
            count_o2_fail = count_o2_fail + 1;
        else
            count_o2_fail = 0;
        end
        isFailed = 0;
    end
else
    isFailed=0;
end
